simulink model "math_model"  (R2024b)
settings: Solver=ode45  StartTime=0.0  StopTime=20  MaxStep=1e-6  RelTol=1e-3
values from neighbouring files (symbols this model uses):
  b1 = 0.2    [compute_pid_from_target.m]    (also in parameters.m)
  b2 = 0.2    [compute_pid_from_target.m]    (also in parameters.m = 1)
  dr_max = 10    [parameters.m]
  dr_min = -10    [parameters.m]
  dtheta_max = 10    [parameters.m]
  dtheta_min = -10    [parameters.m]
  g = 9.8036    [compute_pid_from_target.m]    (also in parameters.m)
  m = 0.01    [compute_pid_from_target.m]    (also in parameters.m = 0.4)
  r_desired = 0.3    [parameters.m]
  r_start = 0.2    [parameters.m]
  rmax = 0.4    [parameters.m]
  rmin = 0.1    [parameters.m]
  theta_desired = pi/2    (= 1.57079632679)    [parameters.m]
  theta_max = pi/2    (= 1.57079632679)    [parameters.m]
  theta_min = -pi/2    (= -1.57079632679)    [parameters.m]
  theta_start = pi/6    (= 0.523598775598)    [parameters.m]
libraries: slpidlib x2
settings Model: Creator=Admin  LastModifiedBy=Admin

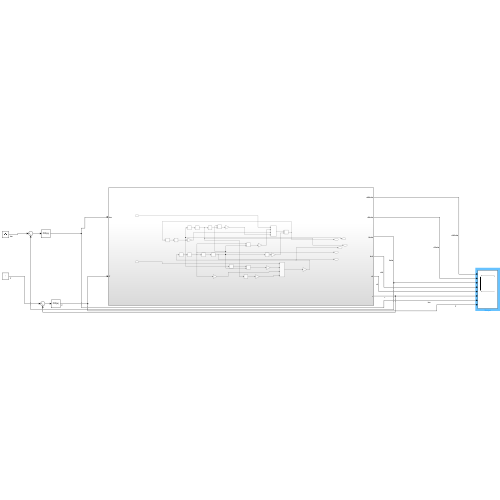
[thumbnail: Simulink's stored preview of the top-level diagram]
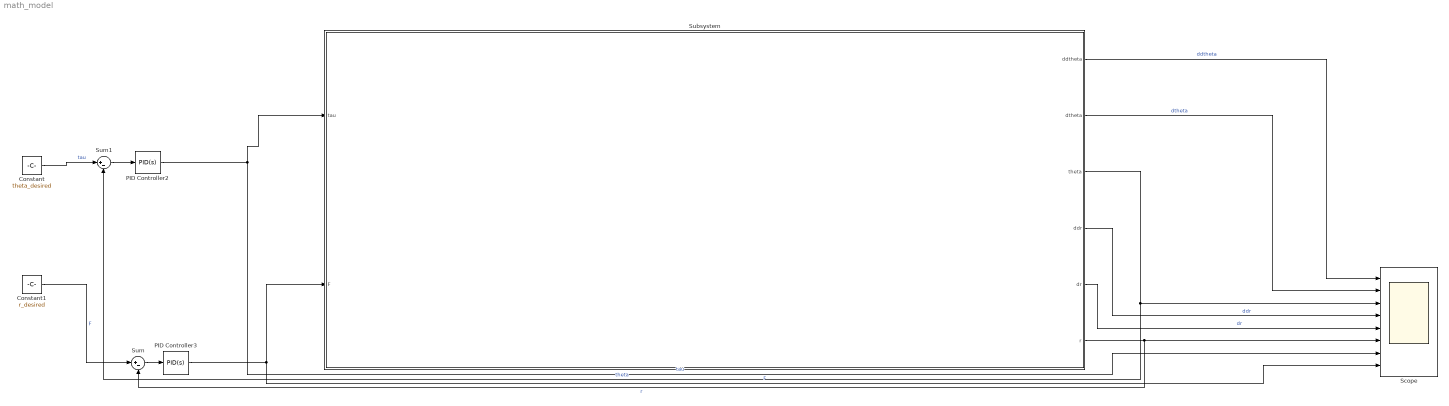
== system math_model ==
  Constant : Constant  Value=theta_desired
  Constant1 : Constant  Value=r_desired
  PID Controller2 : slpidlib/PID Controller  Controller=PID  Form=Parallel  TimeDomain=Continuous-time  UseExternalTs=off  SampleTime=-1  IntegratorMethod=Forward Euler  FilterMethod=Forward Euler  ControllerParametersSource=internal  P=14.6103627720497  I=48.4702036695436  UseKiTs=off  D=0.613140779048183  UseExternalDerivativeSource=off  N=439.327956799177  UseFilter=on  TunerSelectOption=Transfer Function Based (PID Tuner App)  InitialConditionSource=internal  InitialConditionForIntegrator=0  InitialConditionForFilter=0  DifferentiatorICPrevScaledInput=0  ExternalReset=none  TrackingMode=off  Kt=1  LimitOutput=off  SatLimitsSource=internal  UpperSaturationLimit=inf  LowerSaturationLimit=-inf  LinearizeAsGain=on  AntiWindupMode=none  Kb=1  LimitIntegrator=off  UpperIntegratorSaturationLimit=inf  LowerIntegratorSaturationLimit=-inf  POutMin=[]  POutMax=[]  IOutMin=[]  IOutMax=[]  DOutMin=[]  DOutMax=[]  NOutMin=[]  NOutMax=[]  SumOutMin=[]  SumOutMax=[]  SaturationOutMin=[]  SaturationOutMax=[]  PParamMin=[]  PParamMax=[]  IParamMin=[]  IParamMax=[]  DParamMin=[]  DParamMax=[]  NParamMin=[]  NParamMax=[]  KbParamMin=[]  KbParamMax=[]  KtParamMin=[]  KtParamMax=[]  KbOutMin=[]  KbOutMax=[]  KtOutMin=[]  KtOutMax=[]  IntegratorOutMin=[]  IntegratorOutMax=[]  FilterOutMin=[]  FilterOutMax=[]  SumI1OutMin=[]  SumI1OutMax=[]  SumI2OutMin=[]  SumI2OutMax=[]  SumI3OutMin=[]  SumI3OutMax=[]  SumI4OutMin=[]  SumI4OutMax=[]  SumDOutMin=[]  SumDOutMax=[]  DifferentiatorOutMin=[]  DifferentiatorOutMax=[]  FilterDiffOutCoefMin=[]  FilterDiffOutCoefMax=[]  ReciprocalOutMin=[]  ReciprocalOutMax=[]  SumDenOutMin=[]  SumDenOutMax=[]  SumNumOutMin=[]  SumNumOutMax=[]  DivideOutMin=[]  DivideOutMax=[]  UdiffTsProdOutMin=[]  UdiffTsProdOutMax=[]  NTsProdOutMin=[]  NTsProdOutMax=[]  UintegralTsProdOutMin=[]  UintegralTsProdOutMax=[]  UngainTsProdOutMin=[]  UngainTsProdOutMax=[]  ClampingZeroOutDataTypeStr=Inherit: Inherit via back propagation  ClampingZeroOutMin=[]  ClampingZeroOutMax=[]  FilterDenConstantOutDataTypeStr=Inherit: Inherit via back propagation  FilterDenConstantOutMin=[]  FilterDenConstantOutMax=[]  PCopyOutDataTypeStr=Inherit: Inherit via back propagation  PCopyOutMin=[]  PCopyOutMax=[]  NCopyOutDataTypeStr=Inherit: Inherit via back propagation  NCopyOutMin=[]  NCopyOutMax=[]  IntegratorContinuousStateAttributes=''  IntegratorStateMustResolveToSignalObject=off  IntegratorRTWStateStorageClass=Auto  FilterContinuousStateAttributes=''  FilterStateMustResolveToSignalObject=off  FilterRTWStateStorageClass=Auto  ParallelPVariant=InternalParameters  IdealPVariant=Disabled  IVariant=InternalParameters  DVariant=InternalParameters  IntegratorVariant=Continuous  SatVariant=Disabled  AWVariant=Passthrough  PCopyVariant=Disabled  TRVariant=Disabled  FdbkBlocksVariant=Forward  IdealPFdbkVariant=Disabled  SatFdbkVariant=Disabled  DerivativeFilterVariant=ContFilter  NVariant=InternalParameters  NCopyVariant=Disabled  FilterICVariant=InternalICsFilter  IntegratorICVariant=InternalICs  ExternalResetVariant=Disabled  TRSumVariant=Passthrough  SumFdbkVariant=Disabled  SumVariant=Sum_PID  TsampFilterVariant=InternalTs  TsampNgainVariant=Passthrough  TsampIntegralVariant=Disabled_SignalSpec  ExternalSaturationOutDataTypeStr=Inherit: Same as second input  DerivativeSourceVariant=ErrorSignal  PreIntVariant=InternalPreInt
  PID Controller3 : slpidlib/PID Controller  Controller=PID  Form=Parallel  TimeDomain=Continuous-time  UseExternalTs=off  SampleTime=-1  IntegratorMethod=Forward Euler  FilterMethod=Forward Euler  ControllerParametersSource=internal  P=729167.303561147  I=93849952.0734835  UseKiTs=off  D=1043.94594356673  UseExternalDerivativeSource=off  N=14929.1710396329  UseFilter=on  TunerSelectOption=Transfer Function Based (PID Tuner App)  InitialConditionSource=internal  InitialConditionForIntegrator=0  InitialConditionForFilter=0  DifferentiatorICPrevScaledInput=0  ExternalReset=none  TrackingMode=off  Kt=1  LimitOutput=off  SatLimitsSource=internal  UpperSaturationLimit=inf  LowerSaturationLimit=-inf  LinearizeAsGain=on  AntiWindupMode=none  Kb=1  LimitIntegrator=off  UpperIntegratorSaturationLimit=inf  LowerIntegratorSaturationLimit=-inf  POutMin=[]  POutMax=[]  IOutMin=[]  IOutMax=[]  DOutMin=[]  DOutMax=[]  NOutMin=[]  NOutMax=[]  SumOutMin=[]  SumOutMax=[]  SaturationOutMin=[]  SaturationOutMax=[]  PParamMin=[]  PParamMax=[]  IParamMin=[]  IParamMax=[]  DParamMin=[]  DParamMax=[]  NParamMin=[]  NParamMax=[]  KbParamMin=[]  KbParamMax=[]  KtParamMin=[]  KtParamMax=[]  KbOutMin=[]  KbOutMax=[]  KtOutMin=[]  KtOutMax=[]  IntegratorOutMin=[]  IntegratorOutMax=[]  FilterOutMin=[]  FilterOutMax=[]  SumI1OutMin=[]  SumI1OutMax=[]  SumI2OutMin=[]  SumI2OutMax=[]  SumI3OutMin=[]  SumI3OutMax=[]  SumI4OutMin=[]  SumI4OutMax=[]  SumDOutMin=[]  SumDOutMax=[]  DifferentiatorOutMin=[]  DifferentiatorOutMax=[]  FilterDiffOutCoefMin=[]  FilterDiffOutCoefMax=[]  ReciprocalOutMin=[]  ReciprocalOutMax=[]  SumDenOutMin=[]  SumDenOutMax=[]  SumNumOutMin=[]  SumNumOutMax=[]  DivideOutMin=[]  DivideOutMax=[]  UdiffTsProdOutMin=[]  UdiffTsProdOutMax=[]  NTsProdOutMin=[]  NTsProdOutMax=[]  UintegralTsProdOutMin=[]  UintegralTsProdOutMax=[]  UngainTsProdOutMin=[]  UngainTsProdOutMax=[]  ClampingZeroOutDataTypeStr=Inherit: Inherit via back propagation  ClampingZeroOutMin=[]  ClampingZeroOutMax=[]  FilterDenConstantOutDataTypeStr=Inherit: Inherit via back propagation  FilterDenConstantOutMin=[]  FilterDenConstantOutMax=[]  PCopyOutDataTypeStr=Inherit: Inherit via back propagation  PCopyOutMin=[]  PCopyOutMax=[]  NCopyOutDataTypeStr=Inherit: Inherit via back propagation  NCopyOutMin=[]  NCopyOutMax=[]  IntegratorContinuousStateAttributes=''  IntegratorStateMustResolveToSignalObject=off  IntegratorRTWStateStorageClass=Auto  FilterContinuousStateAttributes=''  FilterStateMustResolveToSignalObject=off  FilterRTWStateStorageClass=Auto  ParallelPVariant=InternalParameters  IdealPVariant=Disabled  IVariant=InternalParameters  DVariant=InternalParameters  IntegratorVariant=Continuous  SatVariant=Disabled  AWVariant=Passthrough  PCopyVariant=Disabled  TRVariant=Disabled  FdbkBlocksVariant=Forward  IdealPFdbkVariant=Disabled  SatFdbkVariant=Disabled  DerivativeFilterVariant=ContFilter  NVariant=InternalParameters  NCopyVariant=Disabled  FilterICVariant=InternalICsFilter  IntegratorICVariant=InternalICs  ExternalResetVariant=Disabled  TRSumVariant=Passthrough  SumFdbkVariant=Disabled  SumVariant=Sum_PID  TsampFilterVariant=InternalTs  TsampNgainVariant=Passthrough  TsampIntegralVariant=Disabled_SignalSpec  ExternalSaturationOutDataTypeStr=Inherit: Same as second input  DerivativeSourceVariant=ErrorSignal  PreIntVariant=InternalPreInt
  Scope : Scope  NumInputPorts=8
  Subsystem : Subsystem
  Sum : Sum  Inputs=|+-
  Sum1 : Sum  Inputs=|+-
  wires:
  Subsystem/1(ddtheta) -> Scope/1  "ddtheta"
  Subsystem/2(dtheta) -> Scope/2  "dtheta"
  Subsystem/3(theta) -> Sum1/2, Scope/3  "theta"
  Subsystem/4(ddr) -> Scope/4  "ddr"
  Subsystem/5(dr) -> Scope/5  "dr"
  Subsystem/6(r) -> Sum/2, Scope/6  "r"
  Constant1/1 -> Sum/1  "F"
  Constant/1 -> Sum1/1  "tau"
  Sum/1 -> PID Controller3/1
  PID Controller2/1 -> Subsystem/1(tau), Scope/7  "tau"
  Sum1/1 -> PID Controller2/1
  PID Controller3/1 -> Subsystem/2(F), Scope/8  "F"

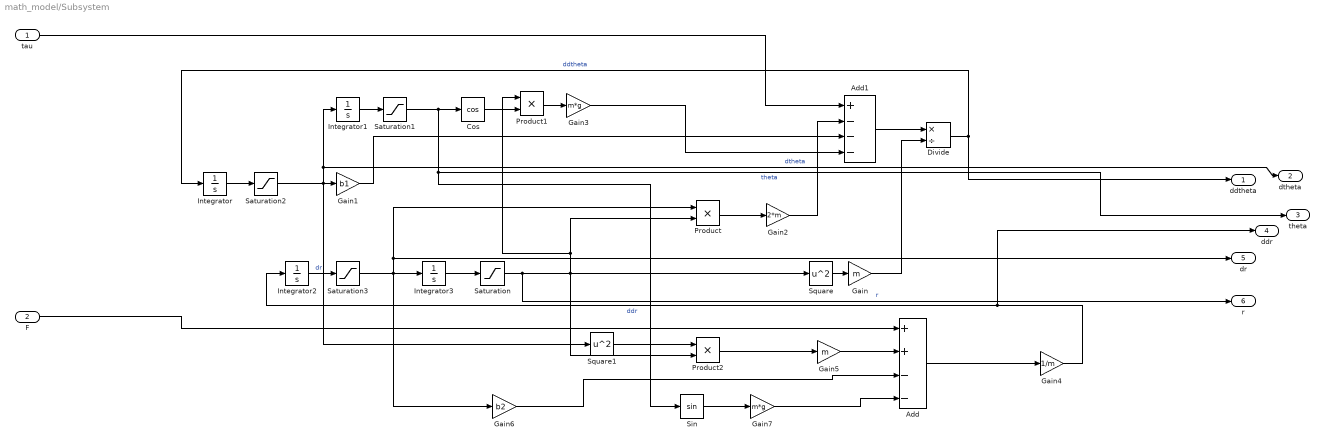
== system math_model/Subsystem ==
  tau : Inport
  F : Inport  Port=2
  Add : Sum  Inputs=++--
  Add1 : Sum  Inputs=+---
  Cos : Trigonometry  Operator=cos
  Divide : Product  Inputs=*/
  Gain : Gain  Gain=m
  Gain1 : Gain  Gain=b1
  Gain2 : Gain  Gain=2*m
  Gain3 : Gain  Gain=m*g
  Gain4 : Gain  Gain=1/m
  Gain5 : Gain  Gain=m
  Gain6 : Gain  Gain=b2
  Gain7 : Gain  Gain=m*g
  Integrator : Integrator
  Integrator1 : Integrator  InitialCondition=theta_start
  Integrator2 : Integrator
  Integrator3 : Integrator  InitialCondition=r_start
  Product : Product
  Product1 : Product
  Product2 : Product
  Saturation : Saturate  UpperLimit=rmax  LowerLimit=rmin
  Saturation1 : Saturate  UpperLimit=theta_max  LowerLimit=theta_min
  Saturation2 : Saturate  UpperLimit=dtheta_max  LowerLimit=dtheta_min
  Saturation3 : Saturate  UpperLimit=dr_max  LowerLimit=dr_min
  Sin : Trigonometry
  Square : Math  Operator=square
  Square1 : Math  Operator=square
  ddtheta : Outport
  dtheta : Outport  Port=2
  theta : Outport  Port=3
  ddr : Outport  Port=4
  dr : Outport  Port=5
  r : Outport  Port=6
  wires:
  Integrator1/1 -> Saturation1/1
  Gain7/1 -> Add/4
  Integrator2/1 -> Saturation3/1  "dr"
  F/1 -> Add/1
  Gain4/1 -> ddr/1, Integrator2/1  "ddr"
  Product2/1 -> Gain5/1
  Saturation2/1 -> dtheta/1, Integrator1/1, Square1/1, Gain1/1  "dtheta"
  Integrator3/1 -> Saturation/1
  Gain5/1 -> Add/2
  tau/1 -> Add1/1
  Saturation1/1 -> theta/1, Sin/1, Cos/1  "theta"
  Divide/1 -> ddtheta/1, Integrator/1  "ddtheta"
  Gain3/1 -> Add1/4
  Saturation/1 -> r/1, Product/2, Product1/1, Product2/2, Square/1  "r"
  Gain6/1 -> Add/3
  Sin/1 -> Gain7/1
  Add/1 -> Gain4/1
  Square1/1 -> Product2/1
  Cos/1 -> Product1/2
  Square/1 -> Gain/1
  Add1/1 -> Divide/1
  Product1/1 -> Gain3/1
  Gain2/1 -> Add1/2
  Product/1 -> Gain2/1
  Gain/1 -> Divide/2
  Gain1/1 -> Add1/3
  Integrator/1 -> Saturation2/1
  Saturation3/1 -> Gain6/1, Product/1, dr/1, Integrator3/1
